simulink model "Ecuaciones_Diferencciales"  (R2017a)
settings: Solver=VariableStepAuto  StartTime=0.0  StopTime=10.0  RelTol=1e-3
settings Model: Creator=Lizeth P. Guzman  LastModifiedBy=Lizeth P. Guzman

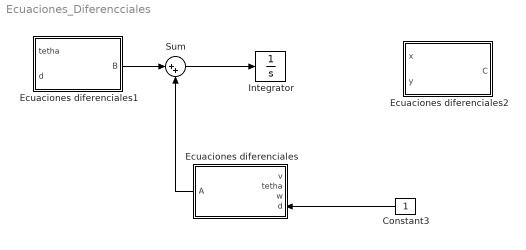
== system Ecuaciones_Diferencciales ==
  Constant3 : Constant
  Ecuaciones diferenciales : MATLAB Function  TreatAsAtomicUnit=on
  Ecuaciones diferenciales1 : MATLAB Function  TreatAsAtomicUnit=on
  Ecuaciones diferenciales2 : MATLAB Function  TreatAsAtomicUnit=on
  Integrator : Integrator
  Sum : Sum  Inputs=|++
  wires:
  Constant3/1 -> Ecuaciones diferenciales/4(d)
  Ecuaciones diferenciales1/1(B) -> Sum/1
  Ecuaciones diferenciales/1(A) -> Sum/2
  Sum/1 -> Integrator/1

== matlab function Ecuaciones_Diferencciales/Ecuaciones diferenciales1 ==
  data: tetha input; B output; d input
function B  = fcn(tetha,d)
%#codegen
d=1;
B=[cos(tetha) -d*sin(tetha);
   sin(tetha)  d*cos(tetha);
   0           1];

== matlab function Ecuaciones_Diferencciales/Ecuaciones diferenciales2 ==
  data: x input; y input; C output
function C  = fcn(x,y)
%#codegen
d=1;
C=[(x)/(((x^2)+(y^2))^(1/2)) (y)/(((x^2)+(y^2))^(1/2)) 0;
    0 0 1 ];

== matlab function Ecuaciones_Diferencciales/Ecuaciones diferenciales ==
  data: v input; tetha input; A output; w input; d input
function A  = fcn(v,tetha,w,d)
%#codegen
d=1;
A=[0 0 -v*sin(tetha)-(d*w*cos(tetha));
   0 0  v*cos(tetha)-(d*w*sin(tetha));
   0 0  0 ];
